simulink library "atmoDrag_lib"  (R2018b)
settings: Solver=VariableStepAuto  StartTime=0.0  StopTime=10.0  RelTol=1e-3
undefined symbols (not defined in the file or in its folder): Earth, simParams, WGS84
libraries: vrlib x1, aerolibtransform2 x1, aerolibatmos2 x1, aerolibutil x1
settings Model: Creator=Kate  LastModifiedBy=colem

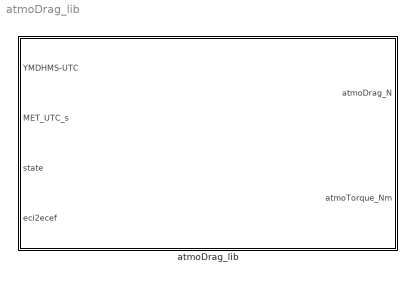
== system atmoDrag_lib ==
  atmoDrag_lib : Subsystem

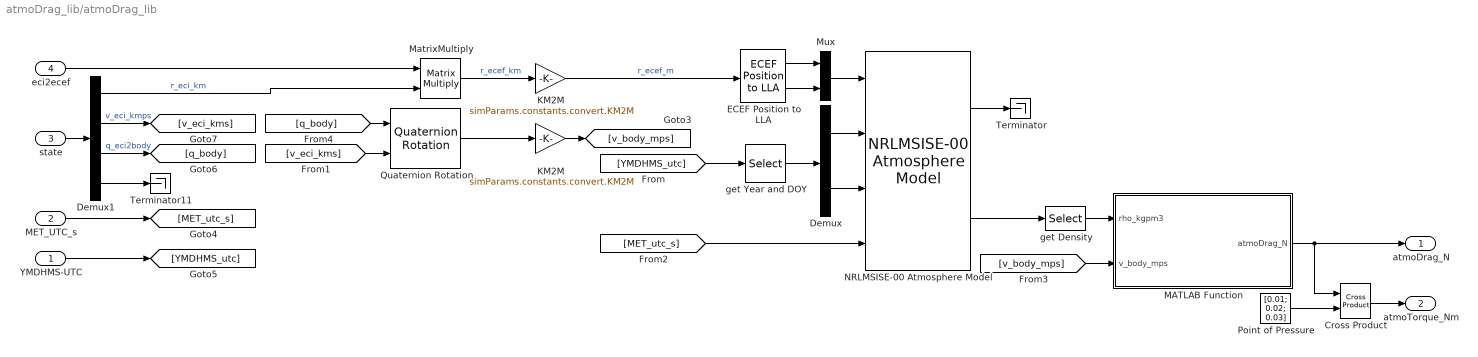
== system atmoDrag_lib/atmoDrag_lib ==
  YMDHMS-UTC : Inport
  MET_UTC_s : Inport  Port=2
  state : Inport  Port=3
  eci2ecef : Inport  Port=4
  Cross Product : vrlib/Utilities/Cross Product
      settings: SourceProductBaseCode=VR
  Demux : Demux  Outputs=[1 1]
  Demux1 : Demux  Outputs=[3 3 4 3]
  ECEF Position to LLA : aerolibtransform2/ECEF Position to LLA  units=Metric (MKS)  ptype=Earth (WGS84)  F=1/298.257223563  R=6378137
      settings: SourceProductName=Aerospace Blockset  SourceProductBaseCode=AE
  KM2M : Gain  Gain=simParams.constants.convert.KM2M
  "KM2M " : Gain  Gain=simParams.constants.convert.KM2M
  MATLAB Function : MATLAB Function  TreatAsAtomicUnit=on
  MatrixMultiply : Product  Multiplication=Matrix(*)
  Mux : Mux  Inputs=[2 1]
  NRLMSISE-00 Atmosphere Model : aerolibatmos2/NRLMSISE-00 Atmosphere Model  units=Metric (MKS)  lst_input=off  flux_ap_input=off  flags_input=Internal  flags=ones(1,23)  oxygen_in=off  action=Warning
      settings: SourceProductName=Aerospace Blockset  SourceProductBaseCode=AE
  Point of Pressure : Constant  Value=[0.01; 0.02; 0.03]
  Quaternion Rotation : aerolibutil/Quaternion Rotation
  Terminator : Terminator
  Terminator11 : Terminator
  get Density : Selector  InputPortWidth=9  IndexOptions=Index vector (dialog)  Indices=6  OutputSizes=1
  get Year and DOY : Selector  InputPortWidth=6  IndexOptions=Index vector (dialog)  Indices=[1 3]  OutputSizes=1
  atmoDrag_N : Outport
  atmoTorque_Nm : Outport  Port=2
  wires:
  Demux/1 -> NRLMSISE-00 Atmosphere Model/2
  Demux/2 -> NRLMSISE-00 Atmosphere Model/3
  get Year and DOY/1 -> Demux/1
  Cross Product/1 -> atmoTorque_Nm/1
  NRLMSISE-00 Atmosphere Model/1 -> Terminator/1
  YMDHMS-UTC/1 -> [YMDHMS_utc]
  NRLMSISE-00 Atmosphere Model/2 -> get Density/1
  MATLAB Function/1(atmoDrag_N) -> Cross Product/1, atmoDrag_N/1
  Point of Pressure/1 -> Cross Product/2
  MET_UTC_s/1 -> [MET_utc_s]
  state/1 -> Demux1/1
  Demux1/4 -> Terminator11/1
  Demux1/1 -> MatrixMultiply/2  "r_eci_km"
  [v_body_mps] -> MATLAB Function/2(v_body_mps)
  Quaternion Rotation/1 -> KM2M/1
  Demux1/3 -> [q_body]  "q_eci2body"
  Demux1/2 -> [v_eci_kms]  "v_eci_kmps"
  "KM2M "/1 -> ECEF Position to LLA/1  "r_ecef_m"
  MatrixMultiply/1 -> "KM2M "/1  "r_ecef_km"
  get Density/1 -> MATLAB Function/1(rho_kgpm3)
  ECEF Position to LLA/1 -> Mux/1
  ECEF Position to LLA/2 -> Mux/2
  Mux/1 -> NRLMSISE-00 Atmosphere Model/1
  KM2M/1 -> [v_body_mps]
  [YMDHMS_utc] -> get Year and DOY/1
  [MET_utc_s] -> NRLMSISE-00 Atmosphere Model/4
  [v_eci_kms] -> Quaternion Rotation/2
  [q_body] -> Quaternion Rotation/1
  eci2ecef/1 -> MatrixMultiply/1

== matlab function atmoDrag_lib/MATLAB Function ==
  data: rho_kgpm3 input; simParams parameter; atmoDrag_N output; v_body_mps input
function atmoDrag_N  = atmoDrag(rho_kgpm3,simParams,v_body_mps)
%Author Kate Williams
%   Date created 2/21/2019
%   function consists of basic atmospheric equations
% 
% References: 
% (1) https://apps.dtic.mil/dtic/tr/fulltext/u2/a285118.pdf pg 16
% (2) http://citeseerx.ist.psu.edu/viewdoc/download?doi=10.1.1.588.3019&rep=rep1&type=pdf
% 
%drag in units of newtons, a 3D vector
%den=density, gathered from density model kg/m^3
%Cd = coeficent of drag, dimensionless
%A=exposed cross sectional area, m^2
%m=mass of cubsat, kg
%vrel= relative velocity m/s^2
%unitV= unit vector of relative velocity


% cubesat parameters
Ax  = simParams.scParams.Ax;
Ay  = simParams.scParams.Ay;
Az  = simParams.scParams.Az;
m   = simParams.scParams.m_2u; 
Cd  = simParams.scParams.CD;  

% magnitude and direction of velocity
vMag    = norm(v_body_mps); % speed
unitV   = v_body_mps./vMag; % direction of the drag

% Compute whetted area -- dot products are the cos(angle) between the unit
% normal of velocity and the body faces. This is the projected area seen
% by an observer looking down the velocity vector direction.
A_ = zeros(3,1); % 3 faces of the s/c can be seen maximum
A_(1) = Ax * dot(unitV,simParams.scParams.xB_dir);
if (A_(1)<0)
    A_(1) = -A_(1);
end
A_(2) = Ay * dot(unitV,simParams.scParams.yB_dir);
if (A_(2)<0)
    A_(2) = -A_(2);
end
A_(3) = Az * dot(unitV,simParams.scParams.zB_dir);
if (A_(3)<0)
    A_(3) = -A_(3);
end
A = sum(A_);

% below drag equation from vallado pg 551 eq8-28 
%   drag occurs in opposite direction of velocity
atmoDrag_N = -(0.5 * rho_kgpm3 * (Cd*A/m) * vMag^2) .* unitV; 

end
